simulink model "MagnetoShield_Calibration_DUE"  (R2019a)
settings: Solver=FixedStepAuto  StartTime=0.0  StopTime=10  RelTol=1e-3  EnableMultiTasking=on
libraries: MagnetoLibrary x2
settings Model: SimulationMode=external  ExtModeTrigDuration=2  Creator=Jakub  LastModifiedBy=jakub
settings OptimizationCC: EnhancedBackFolding=on  PassReuseOutputArgsAs=Individual arguments  MaxStackSize=64  OptimizeBlockOrder=speed  DifferentSizesBufferReuse=on  OptimizationCustomize=off
settings DebuggingCC: ParameterTunabilityLossMsg=error
settings HardwareCC: ProdBitPerPointer=32  ProdBitPerSizeT=32  ProdBitPerPtrDiffT=32  ProdLargestAtomicInteger=Long  ProdLargestAtomicFloat=Double  ProdWordSize=32  ProdHWDeviceType=ARM Compatible->ARM Cortex
settings SFSimCC: MATLABDynamicMemAlloc=off
settings RTWCC: SystemTargetFile=ert.tlc  HardwareBoard=Arduino Due  TLCOptions=-aInlineSetEventsForThisBaseRateFcn=TLC_FALSE -aSuppressMultiTaskScheduler=TLC_FALSE -aRateBasedStepFcn=1  TemplateMakefile=ert_default_tmf  GenerateReport=on  Toolchain=Arduino ARM  BuildConfiguration=Faster Runs  IncludeHyperlinkInReport=on  LaunchReport=on  GenerateTraceInfo=on  GenerateTraceReport=on  GenerateTraceReportSl=on  GenerateTraceReportSf=on  GenerateTraceReportEml=on
settings CodeAppCC: ForceParamTrailComments=on  IgnoreCustomStorageClasses=off  OperatorAnnotations=on  SimulinkDataObjDesc=on  SFDataObjDesc=on  InsertBlockDesc=on
settings ERTTargetCC: SupportContinuousTime=on  SupportVariableSizeSignals=on  ExtModeStaticAllocSize=24576

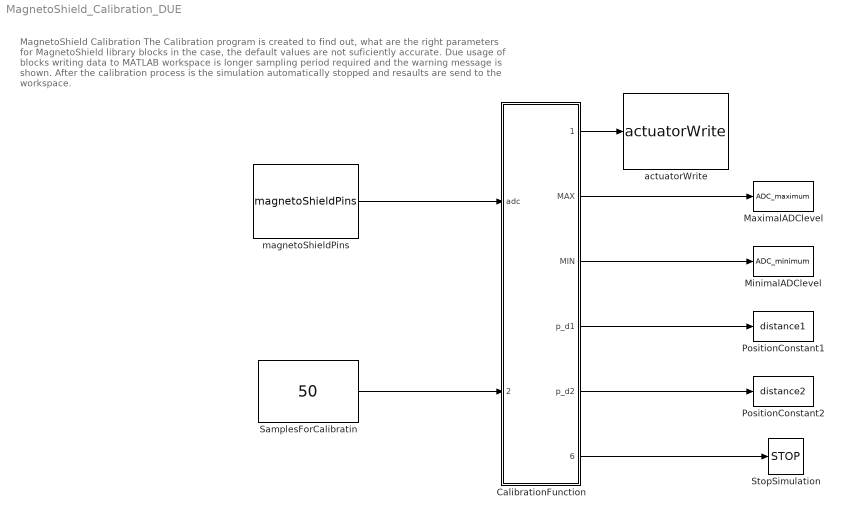
== system MagnetoShield_Calibration_DUE ==
  note: MagnetoShield Calibration
      | The Calibration program is created to find out, what are the right parameters
      | for MagnetoShield library blocks in the case, the default values are not suficiently accurate.
      | Due usage of blocks writing data to MATLAB workspace is longer sampling period required and the warning message is shown.
      | After the calibration process is the simulation automatically stopped and resaults are send to the workspace.
  CalibrationFunction : MATLAB Function  TreatAsAtomicUnit=on
  MaximalADClevel : ToWorkspace  VariableName=ADC_maximum  SampleTime=-1
      settings: MaxDataPoints=1  Save2DSignal=2-D array (concatenate along first dimension)
  MinimalADClevel : ToWorkspace  VariableName=ADC_minimum  SampleTime=-1
      settings: MaxDataPoints=1  Save2DSignal=2-D array (concatenate along first dimension)
  PositionConstant1 : ToWorkspace  VariableName=distance1  SampleTime=-1
      settings: MaxDataPoints=1  Save2DSignal=2-D array (concatenate along first dimension)
  PositionConstant2 : ToWorkspace  VariableName=distance2  SampleTime=-1
      settings: MaxDataPoints=1  Save2DSignal=2-D array (concatenate along first dimension)
  SamplesForCalibratin : Constant  Value=50  SampleTime=0.008
  StopSimulation : Stop
  actuatorWrite : MagnetoLibrary/actuatorWrite  Board=DUE  Units=Volts
      settings: SourceProductName=AutomationShield
  magnetoShieldPins : MagnetoLibrary/magnetoShieldPins  PIN=Hall sensor pin (A3)  sampling=0.008
      settings: SourceProductName=AutomationShield
  wires:
  CalibrationFunction/1(voltage) -> actuatorWrite/1
  CalibrationFunction/2(MAX) -> MaximalADClevel/1
  CalibrationFunction/3(MIN) -> MinimalADClevel/1
  CalibrationFunction/6(terminate) -> StopSimulation/1
  magnetoShieldPins/1 -> CalibrationFunction/1(adc)
  SamplesForCalibratin/1 -> CalibrationFunction/2(samples)
  CalibrationFunction/4(p_d1) -> PositionConstant1/1
  CalibrationFunction/5(p_d2) -> PositionConstant2/1

== matlab function MagnetoShield_Calibration_DUE/CalibrationFunction ==
  data: adc input; voltage output; samples input; MAX output; MIN output; p_d1 output; p_d2 output; terminate output
function [voltage,MAX,MIN,p_d1,p_d2,terminate]  = fcn(adc,samples)
persistent adcMAX adcMIN counter ARES3V3 HALL_SENSITIVITY;
terminate = 0;

if isempty(counter) % inital values of extremes and the counter
    counter = 0;
    adcMAX = 300;
    adcMIN = 300;
    ARES3V3 = 3.3/4095;
    HALL_SENSITIVITY = 769.23;
end

% Minimal ADC level measured on the hall sensor
if counter<=samples
    voltage = 0;
    if adc<adcMIN
        adcMIN = adc;
    end
     MIN = 0;        % outputs of the function during data collection
     MAX = 0;
     p_d1 = 0;
     p_d2 = 0;
% Maximal ADC level measured on the hall sensor
elseif counter>samples && counter<=(2*samples)
    voltage = 12;
    if adc>adcMAX
        adcMAX = adc; 
    end
    MIN = 0;
    MAX = 0;
    p_d1 = 0;
    p_d2 = 0;
% Postprocessing of the measured data and termination of the simulation
else
    voltage = 0;    % Return magnet to the initial position        
    MAX = adcMAX;   % Extrems of ADC levels
    MIN = adcMIN;
    % Constants for position computation in [mm]
    p_d2 = log(17/12)/log((2.5-adcMIN*ARES3V3)*HALL_SENSITIVITY/((2.5-adcMAX*ARES3V3)*HALL_SENSITIVITY));
    p_d1 = 12/((2.5-adcMAX*ARES3V3)*HALL_SENSITIVITY)^p_d2;
    terminate= 1; % terminate simulation
end

counter = counter+1;
end
